simulink model "lyapunovControlLaw"  (R2017b)
settings: Solver=VariableStepAuto  StartTime=0.0  StopTime=time  RelTol=1e-3
values from neighbouring files (symbols this model uses):
  Ktheta = 1    [runLyapunov.m]
  Kx = 1    [runLyapunov.m]
  Ky = 1    [runLyapunov.m]
  L = 0.13    [runDynamic.m]    (also in runLyapunov.m; runStatic.m)
  L_controller = 0.13    [runDynamic.m]    (also in runLyapunov.m = 0.143; runStatic.m)
  R = 2    [runDynamic.m]    (also in runLyapunov.m; runStatic.m)
  r = 0.1    [runDynamic.m]    (also in runLyapunov.m; runStatic.m)
  r_controller = 0.1    [runDynamic.m]    (also in runLyapunov.m; runStatic.m)
  satMax = inf    [runDynamic.m]    (also in runLyapunov.m; runStatic.m)
  satMin = -inf    [runDynamic.m]    (also in runLyapunov.m; runStatic.m)
  thetadInit = pi/2    (= 1.57079632679)    [runLyapunov.m]
  wd = 0.5    [runDynamic.m]    (also in runLyapunov.m; runStatic.m)
  Xi = [2.3; 0; pi]    [runDynamic.m]    (also in runLyapunov.m; runStatic.m)
settings Model: Creator=yleni  LastModifiedBy=yleni

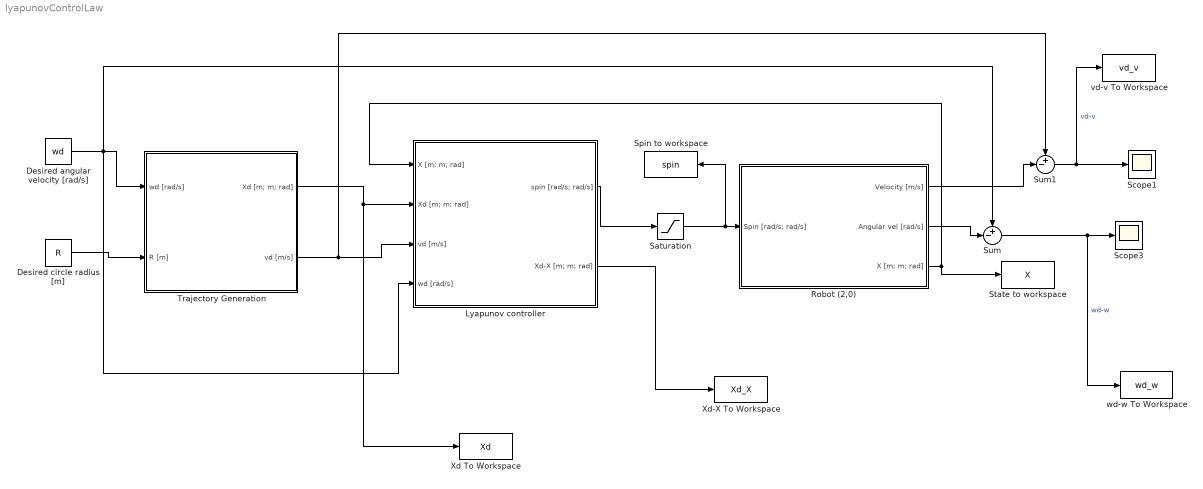
== system lyapunovControlLaw ==
  Desired angular velocity [rad/s] : Constant  Value=wd
  Desired circle radius [m] : Constant  Value=R
  Lyapunov controller : Subsystem  mask{Kx=Kx, Ky=Ky, Ktheta=Ktheta, L=L_controller, r=r_controller}
      mask prompts: Kx "Gain for x position"; Ky "Gain for y position"; Ktheta "Gain for theta orientation"; L "Distance from the wheel to the robot frame center [m]"; r "Wheel radius [m]"
  Robot (2,0) : Subsystem  mask{r=r, L=L, Xstart=Xi}
      mask prompts: r "Wheel radius [m]"; L "Distance from the wheel to the robot frame center [m]"; Xstart "Initial conditions [m; m; rad]"
  Saturation : Saturate  UpperLimit=satMax  LowerLimit=satMin
  Scope1 : Scope
  Scope3 : Scope
  Spin to workspace : ToWorkspace  VariableName=spin  SampleTime=-1
      settings: Save2DSignal=2-D array (concatenate along first dimension)
  State to workspace : ToWorkspace  VariableName=X  SampleTime=-1
      settings: Save2DSignal=2-D array (concatenate along first dimension)
  Sum : Sum  Inputs=+-|
  Sum1 : Sum  Inputs=+-|
  Trajectory Generation : Subsystem  mask{thetaInitial=thetadInit}
      mask prompts: thetaInitial "Initial desired theta [rad]"
  Xd To Workspace : ToWorkspace  VariableName=Xd  SampleTime=-1
      settings: Save2DSignal=2-D array (concatenate along first dimension)
  Xd-X To Workspace : ToWorkspace  VariableName=Xd_X  SampleTime=-1
      settings: Save2DSignal=2-D array (concatenate along first dimension)
  vd-v To Workspace : ToWorkspace  VariableName=vd_v  SampleTime=-1
      settings: Save2DSignal=2-D array (concatenate along first dimension)
  wd-w To Workspace : ToWorkspace  VariableName=wd_w  SampleTime=-1
      settings: Save2DSignal=2-D array (concatenate along first dimension)
  wires:
  Robot (2,0)/3(X [m; m; rad]) -> State to workspace/1, Lyapunov controller/1(X [m; m; rad])
  Desired circle radius [m]/1 -> Trajectory Generation/2(R [m])
  Lyapunov controller/1(spin [rad/s; rad/s]) -> Saturation/1
  Trajectory Generation/1(Xd [m; m; rad]) -> Xd To Workspace/1, Lyapunov controller/2(Xd [m; m; rad])
  Desired angular velocity [rad/s]/1 -> Sum/1, Lyapunov controller/4(wd [rad/s]), Trajectory Generation/1(wd [rad/s])
  Robot (2,0)/2(Angular vel [rad/s]) -> Sum/2
  Sum/1 -> wd-w To Workspace/1, Scope3/1  "wd-w"
  Robot (2,0)/1(Velocity [m/s]) -> Sum1/2
  Sum1/1 -> vd-v To Workspace/1, Scope1/1  "vd-v"
  Trajectory Generation/2(vd [m/s]) -> Sum1/1, Lyapunov controller/3(vd [m/s])
  Saturation/1 -> Spin to workspace/1, Robot (2,0)/1(Spin [rad/s; rad/s])
  Lyapunov controller/2(Xd-X [m; m; rad]) -> Xd-X To Workspace/1

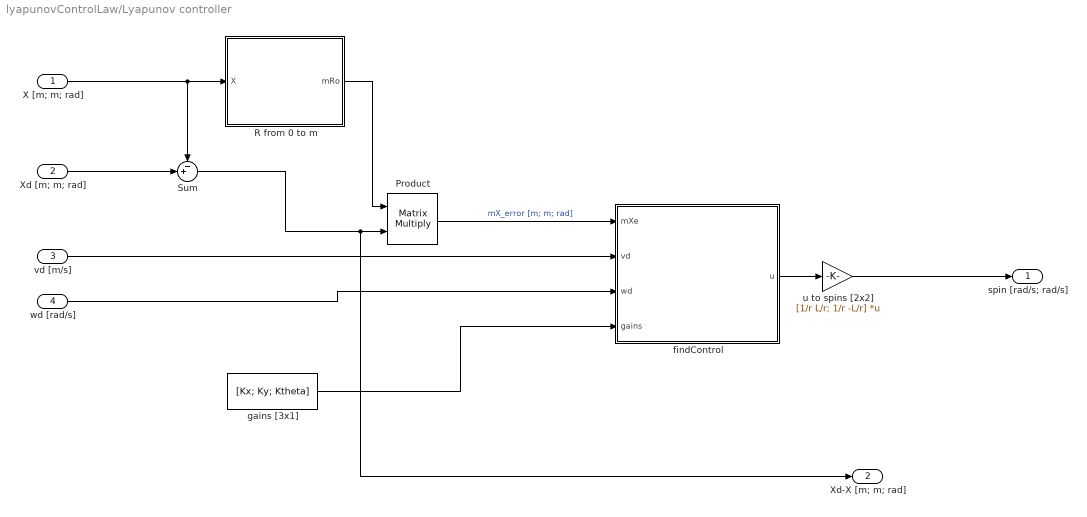
== system lyapunovControlLaw/Lyapunov controller ==
  X [m; m; rad] : Inport
  Xd [m; m; rad] : Inport  Port=2
  vd [m/s] : Inport  Port=3
  wd [rad/s] : Inport  Port=4
  Product : Product  Multiplication=Matrix(*)
  R from 0 to m : MATLAB Function  TreatAsAtomicUnit=on
  Sum : Sum  Inputs=-+|
  findControl : MATLAB Function  TreatAsAtomicUnit=on
  gains [3x1] : Constant  Value=[Kx; Ky; Ktheta]
  u to spins [2x2] : Gain  Gain=[1/r L/r; 1/r -L/r]  Multiplication=Matrix(K*u)
  spin [rad/s; rad/s] : Outport
  Xd-X [m; m; rad] : Outport  Port=2
  wires:
  wd [rad/s]/1 -> findControl/3(wd)
  u to spins [2x2]/1 -> spin [rad/s; rad/s]/1
  X [m; m; rad]/1 -> R from 0 to m/1(X), Sum/1
  vd [m/s]/1 -> findControl/2(vd)
  findControl/1(u) -> u to spins [2x2]/1
  Sum/1 -> Xd-X [m; m; rad]/1, Product/2
  R from 0 to m/1(mRo) -> Product/1
  Product/1 -> findControl/1(mXe)  "mX_error [m; m; rad]"
  Xd [m; m; rad]/1 -> Sum/2
  gains [3x1]/1 -> findControl/4(gains)

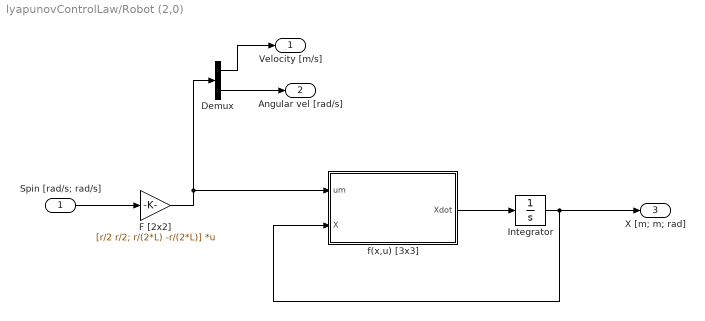
== system lyapunovControlLaw/Robot (2,0) ==
  Spin [rad/s; rad/s] : Inport
  Demux : Demux  Outputs=2
  F [2x2] : Gain  Gain=[r/2 r/2; r/(2*L) -r/(2*L)]  Multiplication=Matrix(K*u)
  Integrator : Integrator  InitialCondition=Xstart
  f(x,u) [3x3] : MATLAB Function  TreatAsAtomicUnit=on
  Velocity [m/s] : Outport
  Angular vel [rad/s] : Outport  Port=2
  X [m; m; rad] : Outport  Port=3
  wires:
  f(x,u) [3x3]/1(Xdot) -> Integrator/1
  F [2x2]/1 -> f(x,u) [3x3]/1(um), Demux/1
  Demux/2 -> Angular vel [rad/s]/1
  Demux/1 -> Velocity [m/s]/1
  Integrator/1 -> X [m; m; rad]/1, f(x,u) [3x3]/2(X)
  Spin [rad/s; rad/s]/1 -> F [2x2]/1

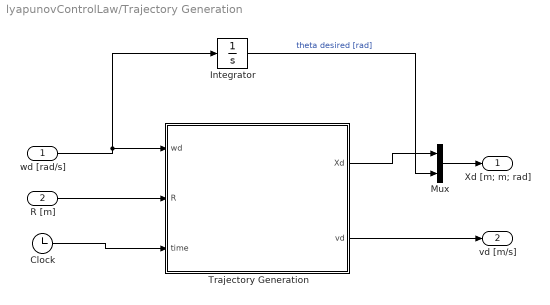
== system lyapunovControlLaw/Trajectory Generation ==
  wd [rad/s] : Inport
  R [m] : Inport  Port=2
  Clock : Clock
  Integrator : Integrator  InitialCondition=thetaInitial
  Mux : Mux  Inputs=2
  Trajectory Generation : MATLAB Function  TreatAsAtomicUnit=on
  Xd [m; m; rad] : Outport
  vd [m/s] : Outport  Port=2
  wires:
  wd [rad/s]/1 -> Integrator/1, Trajectory Generation/1(wd)
  Trajectory Generation/2(vd) -> vd [m/s]/1
  R [m]/1 -> Trajectory Generation/2(R)
  Clock/1 -> Trajectory Generation/3(time)
  Integrator/1 -> Mux/2  "theta desired [rad]"
  Mux/1 -> Xd [m; m; rad]/1
  Trajectory Generation/1(Xd) -> Mux/1

== matlab function lyapunovControlLaw/Lyapunov controller/R from 0 to m ==
  data: X input; mRo output
function mRo = rotationMatrix(X)

mRo = [cos(X(3)) sin(X(3)) 0; -sin(X(3)) cos(X(3)) 0; 0 0 1];

== matlab function lyapunovControlLaw/Robot (2,0)/f(x,u) [3x3] ==
  data: um input; Xdot output; X input
function Xdot  = evolutionModel(um, X)

Xdot = zeros(3,1);
Xdot(1) = um(1) * cos(X(3));
Xdot(2) = um(1) * sin(X(3));
Xdot(3) = um(2);

== matlab function lyapunovControlLaw/Trajectory Generation/Trajectory Generation ==
  data: wd input; Xd output; R input; time input; vd output
function [Xd, vd] = trajectoryGeneration(wd, R, time)

Xd = [R*cos(wd*time); R*sin(wd*time)];

vd = R*wd;

== matlab function lyapunovControlLaw/Lyapunov controller/findControl ==
  data: mXe input; vd input; wd input; u output; gains input
function u = findControl(mXe, vd, wd, gains)

u = [vd * cos(mXe(3)) + gains(1) * mXe(1);
    wd + gains(2) * vd * (sin(mXe(3))/mXe(3)) * mXe(2) + gains(3) * mXe(3)];
